simulink model "capitol2prob5"  (R2013a)
settings: Solver=ode45  StartTime=0.0  StopTime=3600  RelTol=1e-3
undefined symbols (not defined in the file): des, gcbh
settings Model: Creator=user  LastModifiedBy=user

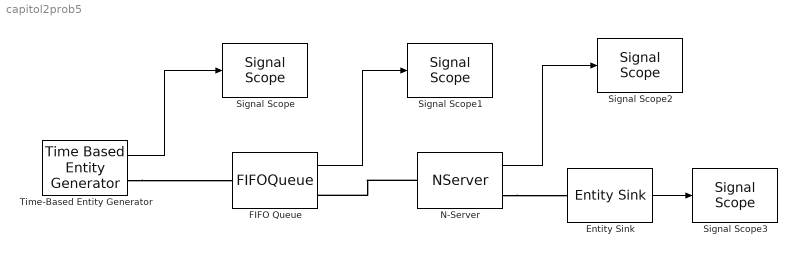
== system capitol2prob5 ==
  Entity Sink : EntitySink  StatNumberArrived=on
  FIFO Queue : FIFOQueue  StatAverageWait=on
      settings: OutputPortMap=o2
  N-Server : NServer  ServiceTime=12  StatNumberInBlock=on
      settings: OutputPortMap=o1
  Signal Scope{,1..3} (4 alike) : SignalScope  LoadFcn=des.scope.CallbackSupport('seLoadFcn',gcbh)  StartFcn=des.scope.CallbackSupport('seStartFcn',gcbh)  StopFcn=des.scope.CallbackSupport('seStopFcn',gcbh)
      settings: CopyFcn=des.scope.CallbackSupport('seCopyFcn',gcbh)  DeleteFcn=des.scope.CallbackSupport('seDeleteFcn',gcbh)  PreSaveFcn=des.scope.CallbackSupport('sePreSaveFcn',gcbh)  NameChangeFcn=des.scope.CallbackSupport('seNameChangeFcn',gcbh)  OpenFcn=des.scope.CallbackSupport('seOpenFcn',gcbh)
  Time-Based Entity Generator : TimeBasedEntityGenerator  Distribution=Exponential  Minimum=12  Maximum=22  Mean=6  StatNumberDeparted=on
  wires:
  Time-Based Entity Generator/1 -> Signal Scope/1
  FIFO Queue/1 -> Signal Scope1/1
  Entity Sink/1 -> Signal Scope3/1
  N-Server/1 -> Signal Scope2/1
  connections:
  Time-Based Entity Generator/RConn1 -- FIFO Queue/LConn1
  N-Server/LConn1 -- FIFO Queue/RConn1
  N-Server/RConn1 -- Entity Sink/LConn1
